simulink model "dampedSystem"  (R2018a)
settings: Solver=VariableStepAuto  StartTime=0.0  StopTime=50  RelTol=1e-3
undefined symbols (not defined in the file): b, k, m
settings Model: Creator=jacks  LastModifiedBy=jacks

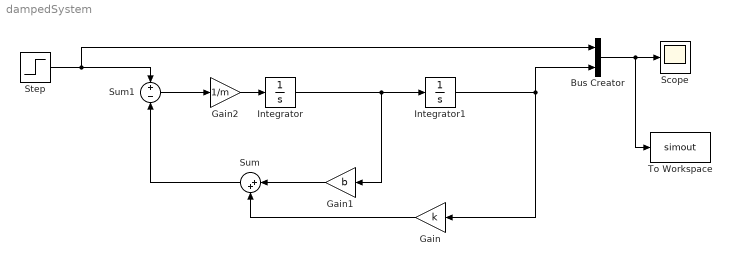
== system dampedSystem ==
  Bus Creator : BusCreator  Inputs=2
  Gain : Gain  Gain=k
  Gain1 : Gain  Gain=b
  Gain2 : Gain  Gain=1/m
  Integrator : Integrator
  Integrator1 : Integrator
  Scope : Scope
  Step : Step  SampleTime=0
  Sum : Sum  Inputs=|++
  Sum1 : Sum  Inputs=+-
  To Workspace : ToWorkspace  VariableName=simout  SaveFormat=Timeseries  SampleTime=-1
  wires:
  Integrator/1 -> Gain1/1, Integrator1/1
  Integrator1/1 -> Bus Creator/2, Gain/1
  Gain1/1 -> Sum/1
  Gain/1 -> Sum/2
  Step/1 -> Bus Creator/1, Sum1/1
  Sum/1 -> Sum1/2
  Sum1/1 -> Gain2/1
  Gain2/1 -> Integrator/1
  Bus Creator/1 -> To Workspace/1, Scope/1
